simulink model "unsolved_solution"  (R2024b)
settings: Solver=VariableStepAuto  StartTime=0.0  StopTime=10.0  RelTol=1e-3
settings Model: Creator=saibot  LastModifiedBy=saibot

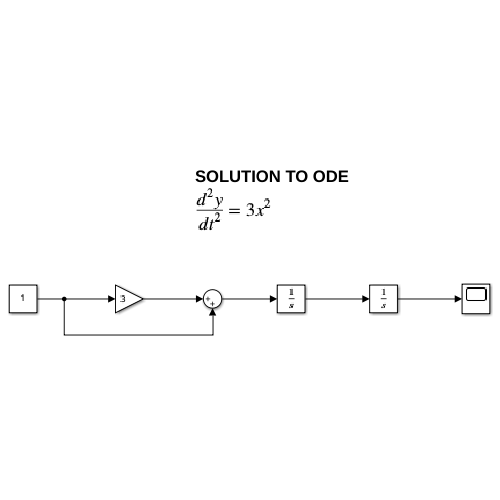
[thumbnail: Simulink's stored preview of the top-level diagram]
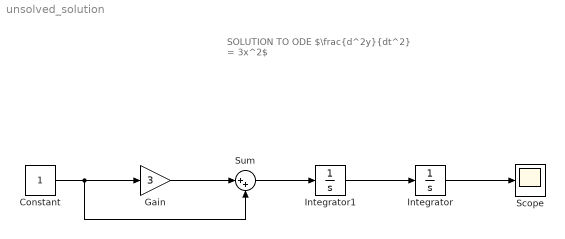
== system unsolved_solution ==
  note: SOLUTION TO ODE
      | $\frac{d^2y}{dt^2} = 3x^2$
  Constant : Constant
  Gain : Gain  Gain=3
  Integrator : Integrator
  Integrator1 : Integrator
  Scope : Scope
  Sum : Sum  Inputs=|++
  wires:
  Sum/1 -> Integrator1/1
  Gain/1 -> Sum/1
  Constant/1 -> Sum/2, Gain/1
  Integrator1/1 -> Integrator/1
  Integrator/1 -> Scope/1
